simulink model "Tavola3_N_FL"  (R2018b)
settings: Solver=FixedStepAuto  StartTime=0.0  StopTime=10  RelTol=1e-3
values from neighbouring files (symbols this model uses):
  cz = R    (= 0.25)    [Again_and_again.m]    (also in Articolo25_NORIPENSAMENTI.m; FeedbackLaw.m; Tavola2.m; Tavola3.m)
  K1 = place(A_min,B_min,poles)    [tavola3_22.m]    (also in tavola3_LAST.m; tavola3_LAST_8_8.m; tavola3_x3x6.m)
  K2 = place(A_min2,B_min2,poles)    [tavola3_22.m]    (also in tavola3_LAST.m; tavola3_LAST_8_8.m; tavola3_x3x6.m)
libraries: simulink x1
settings Model: Creator=Utente  LastModifiedBy=Utente

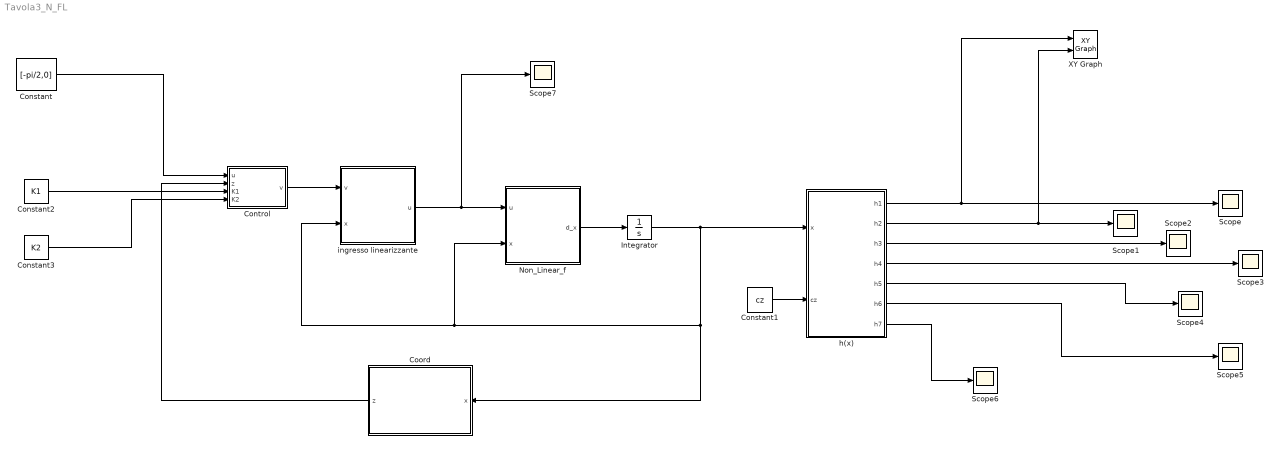
== system Tavola3_N_FL ==
  Constant : Constant  Value=[-pi/2,0]
  Constant1 : Constant  Value=cz
  Constant2 : Constant  Value=K1
  Constant3 : Constant  Value=K2
  Control : MATLAB Function  TreatAsAtomicUnit=on
  Coord : MATLAB Function  TreatAsAtomicUnit=on
  Integrator : Integrator  InitialCondition=[0,0,-pi,0.17,0,5,0]
  "Non_Linear_f " : MATLAB Function  TreatAsAtomicUnit=on
  Scope{,1..7} (8 alike) : Scope
  XY Graph : simulink/Sinks/XY Graph  xmin=-100  xmax=100  ymin=-100  ymax=100  st=-1
  h(x) : MATLAB Function  TreatAsAtomicUnit=on
  ingresso linearizzante : MATLAB Function  TreatAsAtomicUnit=on
  wires:
  "Non_Linear_f "/1(d_x) -> Integrator/1
  Integrator/1 -> Coord/1(x), ingresso linearizzante/2(x), "Non_Linear_f "/2(x), h(x)/1(x)
  h(x)/1(h1) -> XY Graph/1, Scope/1
  ingresso linearizzante/1(u) -> "Non_Linear_f "/1(u), Scope7/1
  Control/1(v) -> ingresso linearizzante/1(v)
  h(x)/2(h2) -> XY Graph/2, Scope1/1
  Constant/1 -> Control/1(u)
  Coord/1(z) -> Control/2(z)
  h(x)/3(h3) -> Scope2/1
  h(x)/4(h4) -> Scope3/1
  h(x)/5(h5) -> Scope4/1
  h(x)/6(h6) -> Scope5/1
  Constant1/1 -> h(x)/2(cz)
  Constant2/1 -> Control/3(K1)
  Constant3/1 -> Control/4(K2)
  h(x)/7(h7) -> Scope6/1

== matlab function Tavola3_N_FL/h(x) ==
  data: x input; h1 output; h2 output; h3 output; h4 output; h5 output; h6 output; h7 output; cz input
function [h1,h2,h3,h4,h5,h6,h7] = h(x,cz)

x1 = x(1);
x2 = x(2);
x3 = x(3);
x4 = x(4);
x5 = x(5);
x6 = x(6);
x7 = x(7);

h1 = x1;
h2 = x2;
h3 = x3;
h4 = x4;
h5 = x5;
h6 = x6;
h7 = x7;

== matlab function Tavola3_N_FL/Non_Linear_f  ==
  data: u input; d_x output; x input
function d_x = statespacef(u,x)

    x1 = x(1);
    x2 = x(2);
    x3 = x(3);
    x4 = x(4);
    x5 = x(5);
    x6 = x(6);
    x7 = x(7);

    f = [                                                                                                                             x6*cos(x3);                                                                                                                            
                                                                                                                                      x6*sin(x3);
                                                                                                                                              x7;
                                                                                                                                              x5;
     (2.39*sin(2.0*x4)*x5^2)/(4.79*cos(x4)^2 - 12.5) - (267.0*sin(x4))/(4.79*cos(x4)^2 - 12.5) - (3.28*x7^2*sin(2.0*x4))/(4.79*cos(x4)^2 - 12.5);
               (1.99*sin(3.0*x4) - 6.77*sin(x4))*x7^2 + (23.5*sin(2.0*x4))/(4.79*cos(x4)^2 - 12.5) - (2.19*x5^2*sin(x4))/(4.79*cos(x4)^2 - 12.5);
                                           (0.547*x6*x7*sin(x4))/(0.228*cos(x4)^2 - 0.315) + (0.228*x5*x7*sin(2.0*x4))/(0.228*cos(x4)^2 - 0.315)];

    g1_b =   [                                          0;
                                                        0;
                                                        0;
                                                        0;
            (2.19*cos(x4) + 3.11)/(4.79*cos(x4)^2 - 12.5);
     -(1.0*(0.547*cos(x4) + 1.0))/(4.79*cos(x4)^2 - 12.5);
                                                        0];

    g2_b = [                           0;
                                       0;
                                       0;
                                       0;
                                       0;
                                       0;
                 -0.05/(0.228*cos(x4)^2 - 0.315)];

    d_x = f + g1_b*u(1) + g2_b*u(2);
    
end

== matlab function Tavola3_N_FL/ingresso linearizzante ==
  data: v input; u output; x input
function u = inputLinearizzante(v,x)

x1 = x(1);
x2 = x(2);
x3 = x(3);
x4 = x(4);
x5 = x(5);
x6 = x(6);
x7 = x(7);

G =  [                                  (0.547*x6*x7*sin(x4))/(0.228*cos(x4)^2 - 0.315) + (0.228*x5*x7*sin(2.0*x4))/(0.228*cos(x4)^2 - 0.315);
 (2.39*sin(2.0*x4)*x5^2)/(4.79*cos(x4)^2 - 12.5) - (267.0*sin(x4))/(4.79*cos(x4)^2 - 12.5) - (3.28*x7^2*sin(2.0*x4))/(4.79*cos(x4)^2 - 12.5)];
 

E = [                                             0, -0.05/(0.228*cos(x4)^2 - 0.315);
     (2.19*cos(x4) + 3.11)/(4.79*cos(x4)^2 - 12.5),                               0];

inv_E = inv(E);

u = -inv_E*G + inv_E*v;

== matlab function Tavola3_N_FL/Coord ==
  data: x input; z output
function z = transformCoordinate(x)

    x1 = x(1);
    x2 = x(2);
    x3 = x(3);
    x4 = x(4);
    x5 = x(5);
    x6 = x(6);
    x7 = x(7);

    z = [   x3;
            x7;
            x4;
            x5;
           -x1;
           -x2;
           -x6];
 

end

== matlab function Tavola3_N_FL/Control ==
  data: u input; z input; v output; K1 input; K2 input
function v = control(u,z,K1,K2)
    
    v = zeros(2,1);
    
    k = [K1(1),K1(2),0,0,0,0,0;
         0,0,K2(1),K2(2),0,0,0];
         
    v(1) = -(k(1,1)*(z(1)-u(1)) + k(1,2)*(z(2)));
    v(2) = -(k(2,3)*(z(3)-u(2)) + k(2,4)*(z(4)));
     
end
